simulink model "complete_plant"  (R2021b)
settings: Solver=VariableStepAuto  StartTime=0.0  StopTime=15  RelTol=1e-3
values from neighbouring files (symbols this model uses):
  a = Simulink.Parameter(1.14)    [startup.m]
  A1 = Simulink.Parameter(39.8344)    [startup.m]
  A2 = Simulink.Parameter(813.0780)    [startup.m]
  b = Simulink.Parameter(-0.03291)    [startup.m]
  B1 = Simulink.Parameter(0.000001287)    [startup.m]
  B2 = Simulink.Parameter(-0.002325)    [startup.m]
  B3 = Simulink.Parameter(3.797)    [startup.m]
  c = Simulink.Parameter(-1.14)    [startup.m]
  C1 = Simulink.Parameter(-0.000000002541)    [startup.m]
  C2 = Simulink.Parameter(0.000005279)    [startup.m]
  C3 = Simulink.Parameter(-0.003943)    [startup.m]
  C4 = Simulink.Parameter(3.634)    [startup.m]
  C_param = Simulink.Parameter([0 13757.41 21278.97 26666.02 30253.47 30313.18 30313.18])    [startup.m]
  d = Simulink.Parameter(-1.027)    [startup.m]
  driver_gain = 1    [startup.m]
  FZ_C = Simulink.Parameter([0 204.13 427.04 668.1 895.72 1124.40 1324.40])    [startup.m]
  gr = Simulink.Parameter([6.63043, 6.63043, 7.95652, 7.95652])    [startup.m]
  I = 15    [startup.m]
  inch2mm = Simulink.Parameter(25.4)    [startup.m]
  J_z = Simulink.Parameter(75)    [startup.m]
  k_limit = Simulink.Parameter(3.461)    [startup.m]
  Ku = Simulink.Parameter(0.24 / g.Value)    [startup.m]
  l = Simulink.Parameter([0.7922471, 0.7828529])    [startup.m]
  max_yaw_field = Simulink.Parameter([1.34 1.34 1.34 1.66 1.14 1.24 0.754 0.849 0.85 0.85])    [startup.m]
  min_speed_regen = Simulink.Parameter(85)    [startup.m]
  motor_efficiency = Simulink.Parameter([0.85, 0.85, 0.85, 0.85])    [startup.m]
  motor_limit_power = Simulink.Parameter([15000, 15000, 15000, 15000])    [startup.m]
  motor_limit_torque = Simulink.Parameter([-25, 25])    [startup.m]
  mu_factor = Simulink.Parameter(2/3)    [startup.m]
  P = 1    [startup.m]
  ramp_rate = 1    [startup.m]
  RE = Simulink.Parameter(0.2228169203)    [startup.m]
  s = Simulink.Parameter([0.647895, 0.62102])    [startup.m]
  S1 = Simulink.Parameter(7 * (10^(-5)))    [startup.m]
  S2 = Simulink.Parameter(-0.0038)    [startup.m]
  S3 = Simulink.Parameter(0.6535)    [startup.m]
  S4 = Simulink.Parameter(0.1061)    [startup.m]
  steer_slope = Simulink.Parameter(0.0111)    [startup.m]
  T = 0    [startup.m]
  T2F = Simulink.Parameter(single([29 29 35 35]))    [startup.m]
  tau = Simulink.Parameter(0)    [startup.m]
  time_delay = 0.022    [startup.m]
  V_target = Simulink.Parameter([0 3 6 9 12 15 18 21 25 31])    [startup.m]
undefined symbols (not defined in the file or in its folder): DiscIntNeverNeededParam
libraries: fl_lib x20, nesl_utility x12, sdl_lib x4, slpidlib x2, simulink x2, autolibdatasheetbattery x1, autolibmappedmotor x1, vehdynlibtire x1, autolibshared x1, vehdynlibviscommon x1
(part 1 of 4)
settings Model: Creator=Inver  LastModifiedBy=Inver
settings DataIOCC: ExternalInput=straight_accel.getElement('driver_input'),straight_accel.getElement('P_A'),straight_accel.getElement('B_A'),straight_accel.getElement('steering_angle'),straight_accel.getElement('batt_temp'),straight_accel.getElement('pressure_front'),straight_accel.getElement('pressure_rear')  LoadExternalInput=on
settings OptimizationCC: DefaultParameterBehavior=Inlined  UseDivisionForNetSlopeComputation=on  GainParamInheritBuiltInType=on  UseFloatMulNetSlope=on  InlineInvariantSignals=on  PassReuseOutputArgsAs=Individual arguments  ZeroExternalMemoryAtStartup=off  ZeroInternalMemoryAtStartup=off  NoFixptDivByZeroProtection=on  EfficientFloat2IntCast=on  LifeSpan=1  OptimizeBlockOrder=speed  DifferentSizesBufferReuse=on  EfficientTunableParamExpr=on
settings DebuggingCC: ParameterTunabilityLossMsg=error
settings HardwareCC: ProdBitPerPointer=32  ProdBitPerSizeT=32  ProdBitPerPtrDiffT=32  ProdLargestAtomicInteger=Long  ProdLargestAtomicFloat=Double  ProdWordSize=32  ProdLongLongMode=on  ProdHWDeviceType=ARM Compatible->ARM Cortex-M
settings SFSimCC: SimCustomHeaderCode="#include \"bigM_v2_func.h\""  SimUserSources=bigM_v2_func.c  MATLABDynamicMemAlloc=off
settings RTWCC: Description=Embedded Coder  SystemTargetFile=ert.tlc  GenCodeOnly=on  TemplateMakefile=ert_default_tmf  BuildConfiguration=Faster Runs
settings CodeAppCC: ForceParamTrailComments=on  IgnoreCustomStorageClasses=off  OperatorAnnotations=on  SimulinkDataObjDesc=on  SFDataObjDesc=on  CustomSymbolStrGlobalVar=rt$N$M  CustomSymbolStrType=$N$M  CustomSymbolStrFcn=$N$M$F  CustomSymbolStrMacro=$N$M  InsertBlockDesc=on
settings ERTTargetCC: TargetLangStandard=C99 (ISO)  GenerateSampleERTMain=on  IncludeMdlTerminateFcn=off  CombineSignalStateStructs=on  SupportComplex=off  SupportNonInlinedSFcns=on  InlinedParameterPlacement=NonHierarchical  ERTCustomFileTemplate=example_file_process.tlc  ERTFilePackagingFormat=CompactWithDataFile

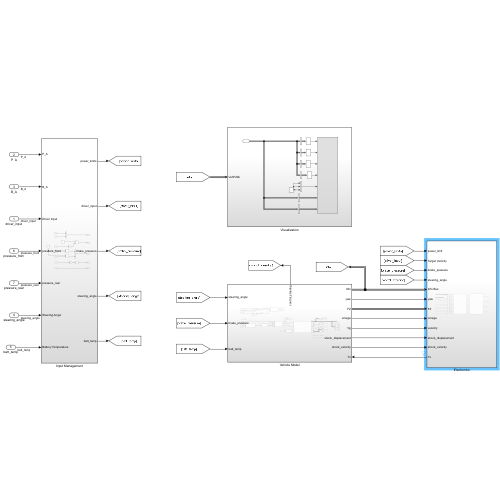
[thumbnail: Simulink's stored preview of the top-level diagram]
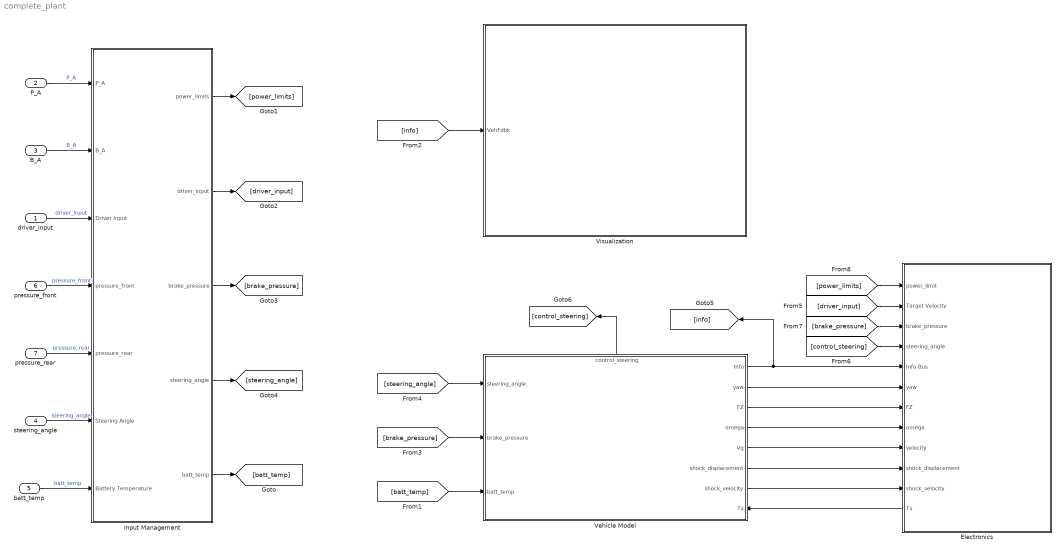
== system complete_plant ==
  driver_input : Inport  Interpolate=off
  P_A : Inport  Port=2  Interpolate=off
  B_A : Inport  Port=3  Interpolate=off
  steering_angle : Inport  Port=4
  batt_temp : Inport  Port=5  Interpolate=off
  pressure_front : Inport  Port=6  Interpolate=off
  pressure_rear : Inport  Port=7  Interpolate=off
  Electronics : Subsystem
      settings: PortSchema="{\"entries\":[{\"content\":{\"sides\":[{\"content\":{\"connectorIds\":[\"In1\",\"In2\",\"In3\",\"In4\",\"In5\",\"In6\",\"In7\",\"In8\",\"In9\",\"In10\",\"In11\",\"Out1\"]},\"type\":\"ConnectorPlacement.EquallySpacedRectSide\",\"uuid\":\"60aa76ce-4868-40a7-a4fe-105a8e1f1745\"},{\"content\":{\"connectorIds\":[],\"side\":\"RIGHT\"},\"type\":\"ConnectorPlacement.EquallySpacedRectSide\",\"uuid\":\"32a33737-884d-4b24-9f96-3d3edd17fbca\"},{\"content\":{\"connectorIds\":[],\"side\":\"TOP\"},\"type\":\"ConnectorPlacement.EquallySpacedRectSide\",\"uuid\":\"827704d2-5b88-4535-b448-6dd72aa29b4b\"},{\"content\":{\"connectorIds\":[],\"side\":\"BOTTOM\"},\"type\":\"ConnectorPlacement.EquallySpacedRectSide\",\"uuid\":\"278cc67c-48ea-4083-b722-927ef88660f9\"},{\"content\":{\"connectorIds\":[],\"side\":\"HIDDEN\"},\"type\":\"ConnectorPlacement.EquallySpacedRectSide\",\"uuid\":\"0c403b58-0099-4716-b0b3-86e3ff44a502\"}]},\"type\":\"ConnectorPlacement.EquallySpacedConnector\",\"uuid\":\"f0e3ee49-9104-4d68-bbfb-d96c82f46588\"}],\"packageUris\":[\"http://schema.mathworks.com/mf0/Connector/R2020b\"],\"version\":\"1.0\"}"
  Input Management : Subsystem
  Vehicle Model : Subsystem
      settings: PortSchema="{\"entries\":[{\"content\":{\"sides\":[{\"content\":{\"connectorIds\":[\"In1\",\"In2\",\"In3\"]},\"type\":\"ConnectorPlacement.EquallySpacedRectSide\",\"uuid\":\"7263df3d-11c2-488e-998f-6bd776306b9c\"},{\"content\":{\"connectorIds\":[\"Out1\",\"Out2\",\"Out3\",\"Out4\",\"Out5\",\"Out6\",\"Out7\",\"In4\"],\"side\":\"RIGHT\"},\"type\":\"ConnectorPlacement.EquallySpacedRectSide\",\"uuid\":\"b0de89c2-35d2-4c59-81fc-f1f509ccf522\"},{\"content\":{\"connectorIds\":[\"Out8\"],\"side\":\"TOP\"},\"type\":\"ConnectorPlacement.EquallySpacedRectSide\",\"uuid\":\"474ba072-8402-41d1-8015-97ca573757b9\"}]},\"type\":\"ConnectorPlacement.EquallySpacedConnector\",\"uuid\":\"426f55ca-7f3f-41f0-94e6-91e6d6304a5e\"}],\"packageUris\":[\"http://schema.mathworks.com/mf0/Connector/R2020b\"],\"version\":\"1.0\"}"
  Visualization : Subsystem
  wires:
  Vehicle Model/5(Vg) -> Electronics/9(velocity)
  Vehicle Model/4(omega) -> Electronics/8(omega)
  [brake_pressure] -> Vehicle Model/2(brake_pressure)
  Vehicle Model/1(Info) -> [info], Electronics/5(Info Bus)
  Vehicle Model/3(FZ) -> Electronics/7(FZ)
  Vehicle Model/2(yaw) -> Electronics/6(yaw)
  Vehicle Model/6(shock_displacement) -> Electronics/10(shock_displacement)
  Vehicle Model/7(shock_velocity) -> Electronics/11(shock_velocity)
  [batt_temp] -> Vehicle Model/3(batt_temp)
  steering_angle/1 -> Input Management/6(Steering Angle)  "steering_angle"
  driver_input/1 -> Input Management/3(Driver Input)  "driver_input"
  P_A/1 -> Input Management/1(P_A)  "P_A"
  pressure_front/1 -> Input Management/4(pressure_front)  "pressure_front"
  B_A/1 -> Input Management/2(B_A)  "B_A"
  pressure_rear/1 -> Input Management/5(pressure_rear)  "pressure_rear"
  batt_temp/1 -> Input Management/7(Battery Temperature)  "batt_temp"
  Input Management/5(batt_temp) -> [batt_temp]
  Input Management/4(steering_angle) -> [steering_angle]
  Input Management/3(brake_pressure) -> [brake_pressure]
  Input Management/2(driver_input) -> [driver_input]
  Input Management/1(power_limits) -> [power_limits]
  [power_limits] -> Electronics/1(power_limit)
  [driver_input] -> Electronics/2(Target Velocity)
  [brake_pressure] -> Electronics/3(brake_pressure)
  [control_steering] -> Electronics/4(steering_angle)
  [steering_angle] -> Vehicle Model/1(steering_angle)
  [info] -> Visualization/1(VehFdbk)
  Electronics/1(Tx) -> Vehicle Model/4(Tx)
  Vehicle Model/8(control_steering) -> [control_steering]

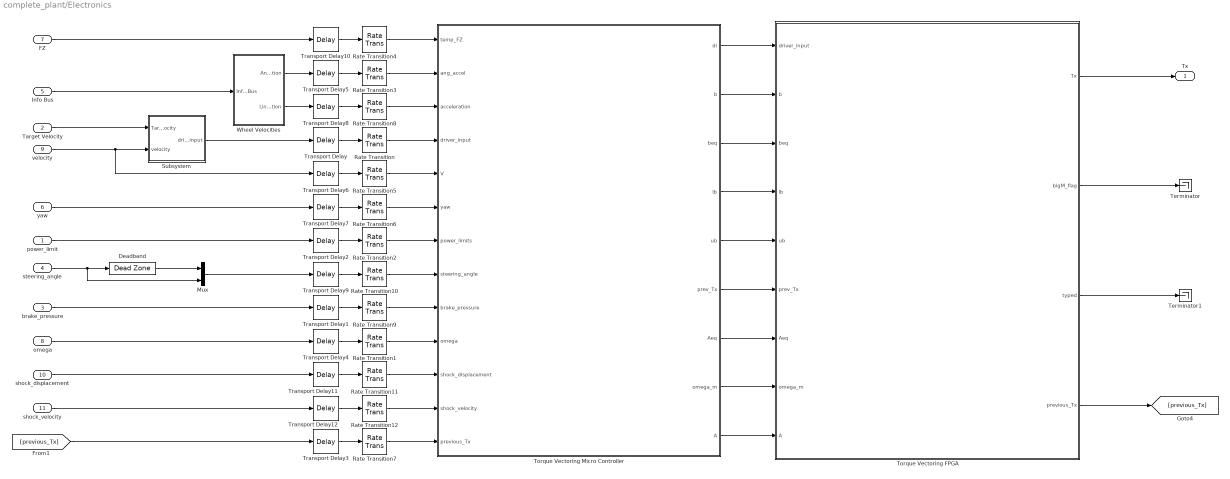
== system complete_plant/Electronics ==
  power_limit : Inport
  Target Velocity : Inport  Port=2
  brake_pressure : Inport  Port=3  PortDimensions=[1 4]
  steering_angle : Inport  Port=4
  Info Bus : Inport  Port=5
  yaw : Inport  Port=6
  FZ : Inport  Port=7
  omega : Inport  Port=8
  velocity : Inport  Port=9
  shock_displacement : Inport  Port=10
  shock_velocity : Inport  Port=11
  " Wheel Velocities" : Subsystem
  Deadband : DeadZone  LowerValue=-3  UpperValue=3  SaturateOnIntegerOverflow=on
  Mux : Mux  Inputs=2
  Rate Transition : RateTransition  OutPortSampleTime=0.015
  Rate Transition{1,7,9,11..12} (5 alike) : RateTransition  InitialCondition=[0 0 0 0]  OutPortSampleTime=0.015
  Rate Transition{2,5,8,10} (4 alike) : RateTransition  InitialCondition=[0 0]  OutPortSampleTime=0.015
  Rate Transition3 : RateTransition  OutPortSampleTime=0.015
  Rate Transition4 : RateTransition  InitialCondition=[450 450 450 450]  OutPortSampleTime=0.015
  Rate Transition6 : RateTransition  OutPortSampleTime=0.015
  Subsystem : Subsystem
  Terminator : Terminator
  Terminator1 : Terminator
  Torque Vectoring FPGA : Subsystem
  Torque Vectoring Micro Controller : Subsystem
  Transport Delay : TransportDelay  DelayTime=time_delay  BufferSize=25000
  Transport Delay{1,3..4,11..12} (5 alike) : TransportDelay  DelayTime=time_delay  InitialOutput=[0 0 0 0]  BufferSize=25000
  Transport Delay10 : TransportDelay  DelayTime=time_delay  InitialOutput=[450 450 450 450]  BufferSize=25000
  Transport Delay{2,6,8..9} (4 alike) : TransportDelay  DelayTime=time_delay  InitialOutput=[0 0]  BufferSize=25000
  Transport Delay5 : TransportDelay  DelayTime=time_delay  BufferSize=25000
  Transport Delay7 : TransportDelay  DelayTime=time_delay  BufferSize=25000
  Tx : Outport  PortDimensions=[1 4]
  wires:
  Info Bus/1 -> " Wheel Velocities"/1(Info Bus)
  Transport Delay6/1 -> Rate Transition5/1
  Transport Delay2/1 -> Rate Transition2/1
  power_limit/1 -> Transport Delay2/1
  Transport Delay7/1 -> Rate Transition6/1
  Transport Delay10/1 -> Rate Transition4/1
  FZ/1 -> Transport Delay10/1
  Subsystem/1(driver_input) -> Transport Delay/1
  yaw/1 -> Transport Delay7/1
  velocity/1 -> Transport Delay6/1, Subsystem/2(velocity)
  Target Velocity/1 -> Subsystem/1(Target Velocity)
  Rate Transition4/1 -> Torque Vectoring Micro Controller/1(temp_FZ)
  Rate Transition6/1 -> Torque Vectoring Micro Controller/6(yaw)
  Rate Transition/1 -> Torque Vectoring Micro Controller/4(driver_input)
  Transport Delay1/1 -> Rate Transition9/1
  brake_pressure/1 -> Transport Delay1/1
  Transport Delay9/1 -> Rate Transition10/1
  Rate Transition10/1 -> Torque Vectoring Micro Controller/8(steering_angle)
  Torque Vectoring FPGA/2(bigM_flag) -> Terminator/1
  Torque Vectoring FPGA/3(typed) -> Terminator1/1
  Rate Transition5/1 -> Torque Vectoring Micro Controller/5(V)
  Rate Transition2/1 -> Torque Vectoring Micro Controller/7(power_limits)
  Transport Delay5/1 -> Rate Transition3/1
  Rate Transition3/1 -> Torque Vectoring Micro Controller/2(ang_accel)
  " Wheel Velocities"/1(Angular Acceleration) -> Transport Delay5/1
  Transport Delay/1 -> Rate Transition/1
  Transport Delay4/1 -> Rate Transition1/1
  Transport Delay11/1 -> Rate Transition11/1
  Transport Delay12/1 -> Rate Transition12/1
  omega/1 -> Transport Delay4/1
  shock_displacement/1 -> Transport Delay11/1
  shock_velocity/1 -> Transport Delay12/1
  Torque Vectoring FPGA/1(Tx) -> Tx/1
  Torque Vectoring Micro Controller/1(di) -> Torque Vectoring FPGA/1(driver_input)
  Torque Vectoring Micro Controller/2(b) -> Torque Vectoring FPGA/2(b)
  Torque Vectoring Micro Controller/3(beq) -> Torque Vectoring FPGA/3(beq)
  Torque Vectoring Micro Controller/4(lb) -> Torque Vectoring FPGA/4(lb)
  Torque Vectoring Micro Controller/8(omega_m) -> Torque Vectoring FPGA/8(omega_m)
  Torque Vectoring Micro Controller/7(Aeq) -> Torque Vectoring FPGA/7(Aeq)
  Torque Vectoring Micro Controller/6(prev_Tx) -> Torque Vectoring FPGA/6(prev_Tx)
  Torque Vectoring Micro Controller/9(A) -> Torque Vectoring FPGA/9(A)
  Torque Vectoring FPGA/4(previous_Tx) -> [previous_Tx]
  Transport Delay3/1 -> Rate Transition7/1
  [previous_Tx] -> Transport Delay3/1
  Rate Transition9/1 -> Torque Vectoring Micro Controller/9(brake_pressure)
  Rate Transition1/1 -> Torque Vectoring Micro Controller/10(omega)
  Rate Transition11/1 -> Torque Vectoring Micro Controller/11(shock_displacement)
  Rate Transition12/1 -> Torque Vectoring Micro Controller/12(shock_velocity)
  Rate Transition7/1 -> Torque Vectoring Micro Controller/13(previous_Tx)
  Torque Vectoring Micro Controller/5(ub) -> Torque Vectoring FPGA/5(ub)
  Transport Delay8/1 -> Rate Transition8/1
  Rate Transition8/1 -> Torque Vectoring Micro Controller/3(acceleration)
  " Wheel Velocities"/2(Linear Acceleration) -> Transport Delay8/1
  steering_angle/1 -> Mux/2, Deadband/1
  Deadband/1 -> Mux/1
  Mux/1 -> Transport Delay9/1

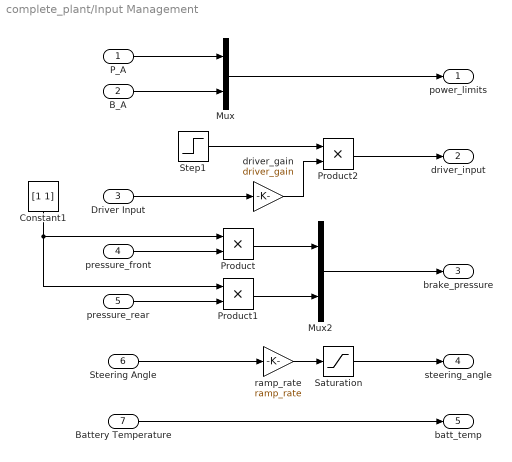
== system complete_plant/Input Management ==
  P_A : Inport
  B_A : Inport  Port=2
  Driver Input : Inport  Port=3
  pressure_front : Inport  Port=4
  pressure_rear : Inport  Port=5
  Steering Angle : Inport  Port=6
  Battery Temperature : Inport  Port=7
  Constant1 : Constant  Value=[1 1]  VectorParams1D=off
  Mux : Mux  Inputs=2
  Mux2 : Mux  Inputs=2
  Product : Product
  Product1 : Product
  Product2 : Product
  Saturation : Saturate  UpperLimit=30  LowerLimit=-30
  Step1 : Step  Time=0.05  SampleTime=0
  driver_gain : Gain  Gain=driver_gain
  ramp_rate : Gain  Gain=ramp_rate
  power_limits : Outport
  driver_input : Outport  Port=2
  brake_pressure : Outport  Port=3
  steering_angle : Outport  Port=4
  batt_temp : Outport  Port=5
  wires:
  ramp_rate/1 -> Saturation/1
  Steering Angle/1 -> ramp_rate/1
  Driver Input/1 -> driver_gain/1
  Mux/1 -> power_limits/1
  P_A/1 -> Mux/1
  B_A/1 -> Mux/2
  Saturation/1 -> steering_angle/1
  pressure_front/1 -> Product/2
  Battery Temperature/1 -> batt_temp/1
  Product/1 -> Mux2/1
  Product1/1 -> Mux2/2
  Mux2/1 -> brake_pressure/1
  Constant1/1 -> Product1/1, Product/1
  pressure_rear/1 -> Product1/2
  Step1/1 -> Product2/1
  driver_gain/1 -> Product2/2
  Product2/1 -> driver_input/1

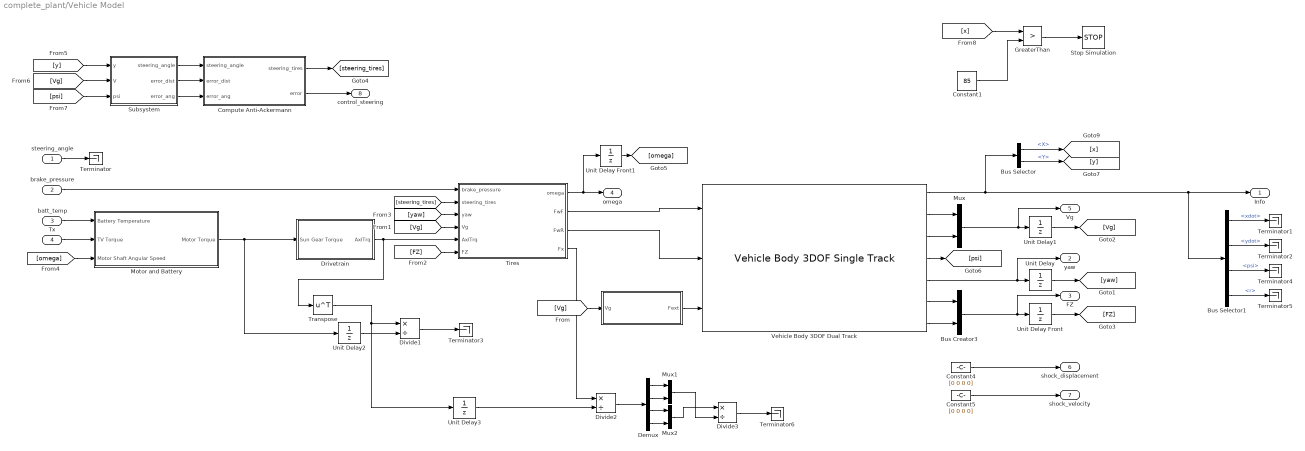
== system complete_plant/Vehicle Model ==
  steering_angle : Inport
  brake_pressure : Inport  Port=2
  batt_temp : Inport  Port=3
  Tx : Inport  Port=4
  "  " : MATLAB Function  TreatAsAtomicUnit=on  SystemSampleTime=0.0005
  Bus Creator3 : BusCreator  Inputs=2
  Bus Selector : BusSelector  OutputSignals=InertFrm.Cg.Disp.X,InertFrm.Cg.Disp.Y
  Bus Selector1 : BusSelector  OutputSignals=BdyFrm.Cg.Vel.xdot,BdyFrm.Cg.Vel.ydot,InertFrm.Cg.Ang.psi,BdyFrm.Cg.AngVel.r
  Compute Anti-Ackermann : MATLAB Function  TreatAsAtomicUnit=on  SystemSampleTime=0.0005
  Constant1 : Constant  Value=85
  Constant4 : Constant  Value=[0 0 0 0]
  Constant5 : Constant  Value=[0 0 0 0]
  Demux : Demux
  Divide1 : Product  Inputs=*/
  Divide2 : Product  Inputs=*/
  Divide3 : Product  Inputs=*/
  Drivetrain : Subsystem
  GreaterThan : RelationalOperator  Operator=>  OutDataTypeStr=boolean  RndMeth=Simplest
  Motor and Battery : Subsystem
      settings: PortSchema="{\"entries\":[{\"content\":{\"sides\":[{\"content\":{\"connectorIds\":[\"Out1\"]},\"type\":\"ConnectorPlacement.EquallySpacedRectSide\",\"uuid\":\"0a1f914b-70eb-46fa-9e3d-552685e5145b\"},{\"content\":{\"connectorIds\":[\"In1\",\"In2\",\"In3\"],\"side\":\"RIGHT\"},\"type\":\"ConnectorPlacement.EquallySpacedRectSide\",\"uuid\":\"3f4913ad-53b1-4c2d-9942-63851d66d84d\"},{\"content\":{\"connectorIds\":[],\"side\":\"TOP\"},\"type\":\"ConnectorPlacement.EquallySpacedRectSide\",\"uuid\":\"355326fa-9c02-45e7-a319-d2a0d6b3d4bd\"},{\"content\":{\"connectorIds\":[],\"side\":\"HIDDEN\"},\"type\":\"ConnectorPlacement.EquallySpacedRectSide\",\"uuid\":\"65af7ff0-f0aa-4be0-a188-dc3dcb8956e6\"}]},\"type\":\"ConnectorPlacement.EquallySpacedConnector\",\"uuid\":\"023a46d9-a637-4c8e-84c1-6893dcef87c2\"}],\"packageUris\":[\"http://schema.mathworks.com/mf0/Connector/R2020b\"],\"version\":\"1.0\"}"
  Mux : Mux  Inputs=2
  Mux1 : Mux  Inputs=2
  Mux2 : Mux  Inputs=2
  Stop Simulation : Stop
  Subsystem : Subsystem
  Terminator{,1..6} (7 alike) : Terminator
  Tires : Subsystem
  Transpose : Math  Operator=transpose  SaturateOnIntegerOverflow=on
  Unit Delay : UnitDelay  SampleTime=0.0005  HasFrameUpgradeWarning=on
  Unit Delay Front : UnitDelay  InitialCondition=[450 450 450 450]  SampleTime=0.0005  HasFrameUpgradeWarning=on
  Unit Delay Front1 : UnitDelay  InitialCondition=[0 0 0 0]  SampleTime=0.0005  HasFrameUpgradeWarning=on
  Unit Delay1 : UnitDelay  InitialCondition=[0.1 0.1]  SampleTime=0.0005  HasFrameUpgradeWarning=on
  Unit Delay2 : UnitDelay  InitialCondition=[0 0 0 0]  SampleTime=0.0005  HasFrameUpgradeWarning=on
  Unit Delay3 : UnitDelay  InitialCondition=[0 0 0 0]  SampleTime=0.0005  HasFrameUpgradeWarning=on
  Vehicle Body 3DOF Dual Track : autolibshared/Vehicle Body 3DOF Single Track  trackMode=Dual  inputMode=External forces  frontSteerMode=off  rearSteerMode=off  windMode=off  muMode=off  extFMode=on  extMMode=off  htchFMode=off  htchMMode=off  extXo=off  extpsio=off  extxdoto=off  extro=off  extYo=off  extTamb=off  extydoto=off  aMode=2  NF=2  NR=2  m=308  a=0.7922471  b=0.7828529  h=0.295  dh=1  hh=0.2  X_o=0  xdot_o=0  CalphaMode=off  sigmaMode=on  d=0  hl=0  w=[1.29579,1.24204]  Cy_f=25e3  Cy_r=25e3  sigma_f=.1  sigma_r=.1  alpha_f_brk=[-.1 .1]  Cy_f_data=[-9e3 9e3]  alpha_r_brk=[-.1 .1]  Cy_r_data=[-9e3 9e3]  Y_o=0  ydot_o=0  Izz=200  psi_o=0  r_o=0  Af=1.0221  Cd=1.149  Cl=0  Cpm=.00000001  beta_w=[0:0.01:0.1]  Cs=[0:0.0000001:0.000001]  Cym=[0:0.0000001:0.000001]  Pabs=101325  Tair=273  g=9.81  mu=1  xdot_tol=.001  Fznom=15000  Fxtire_sat=7e4  Fytire_sat=7e4  longOff=0  latOff=0  vertOff=0  wrapAng=off
      settings: SourceProductBaseCode=PW,DR,MT,UV,VE
  Info : Outport
  yaw : Outport  Port=2
  FZ : Outport  Port=3
  omega : Outport  Port=4
  Vg : Outport  Port=5
  shock_displacement : Outport  Port=6
  shock_velocity : Outport  Port=7
  control_steering : Outport  Port=8
  wires:
  Vehicle Body 3DOF Dual Track/1 -> Bus Selector/1, Bus Selector1/1, Info/1
  Bus Selector/1 -> [x]  "<X>"
  Bus Selector/2 -> [y]  "<Y>"
  Vehicle Body 3DOF Dual Track/7 -> Bus Creator3/2
  Vehicle Body 3DOF Dual Track/6 -> Bus Creator3/1
  "  "/1(Fext) -> Vehicle Body 3DOF Dual Track/3
  Bus Creator3/1 -> Unit Delay Front/1, FZ/1
  Vehicle Body 3DOF Dual Track/3 -> Mux/2
  Vehicle Body 3DOF Dual Track/2 -> Mux/1
  Mux/1 -> Unit Delay1/1, Vg/1
  Vehicle Body 3DOF Dual Track/5 -> Unit Delay/1, yaw/1
  Unit Delay1/1 -> [Vg]
  Unit Delay/1 -> [yaw]
  [Vg] -> "  "/1(Vg)
  Unit Delay Front/1 -> [FZ]
  brake_pressure/1 -> Tires/1(brake_pressure)
  Tires/1(omega) -> omega/1, Unit Delay Front1/1
  [FZ] -> Tires/6(FZ)
  [steering_tires] -> Tires/2(steering_tires)
  Tires/2(FwF) -> Vehicle Body 3DOF Dual Track/1
  Tires/3(FwR) -> Vehicle Body 3DOF Dual Track/2
  [Vg] -> Tires/4(Vg)
  [yaw] -> Tires/3(yaw)
  Constant5/1 -> shock_velocity/1
  Constant4/1 -> shock_displacement/1
  Unit Delay Front1/1 -> [omega]
  [omega] -> Motor and Battery/1(Motor Shaft Angular Speed)
  batt_temp/1 -> Motor and Battery/3(Battery Temperature)
  Vehicle Body 3DOF Dual Track/4 -> [psi]
  Motor and Battery/1(Motor Torque) -> Drivetrain/1(Sun Gear Torque), Unit Delay2/1
  steering_angle/1 -> Terminator/1
  Bus Selector1/1 -> Terminator1/1  "<xdot>"
  Bus Selector1/2 -> Terminator2/1  "<ydot>"
  Bus Selector1/3 -> Terminator4/1  "<psi>"
  Bus Selector1/4 -> Terminator5/1  "<r>"
  Tx/1 -> Motor and Battery/2(TV Torque)
  Compute Anti-Ackermann/1(steering_tires) -> [steering_tires]
  Compute Anti-Ackermann/2(error) -> control_steering/1
  GreaterThan/1 -> Stop Simulation/1
  [x] -> GreaterThan/1
  Constant1/1 -> GreaterThan/2
  Divide1/1 -> Terminator3/1
  Divide2/1 -> Demux/1
  Tires/4(Fx) -> Divide2/1
  Demux/1 -> Mux1/1
  Demux/2 -> Mux1/2
  Demux/4 -> Mux2/2
  Demux/3 -> Mux2/1
  Mux1/1 -> Divide3/2
  Mux2/1 -> Divide3/1
  Divide3/1 -> Terminator6/1
  Transpose/1 -> Unit Delay3/1, Divide1/1
  Drivetrain/1(AxlTrq) -> Transpose/1, Tires/5(AxlTrq)
  Unit Delay2/1 -> Divide1/2
  Unit Delay3/1 -> Divide2/2
  [y] -> Subsystem/1(y)
  [Vg] -> Subsystem/2(V)
  [psi] -> Subsystem/3(psi)
  Subsystem/1(steering_angle) -> Compute Anti-Ackermann/1(steering_angle)
  Subsystem/2(error_dist) -> Compute Anti-Ackermann/2(error_dist)
  Subsystem/3(error_ang) -> Compute Anti-Ackermann/3(error_ang)

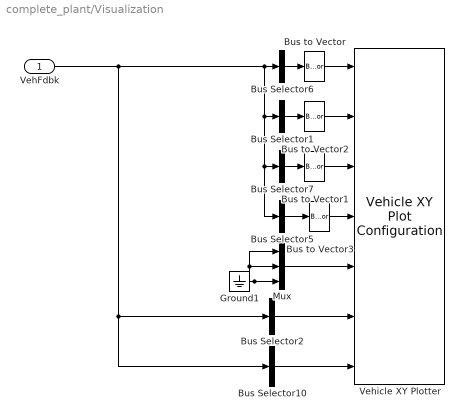
== system complete_plant/Visualization ==
  VehFdbk : Inport
  Bus Selector1 : BusSelector  OutputSignals=InertFrm.Cg.Ang.phi,InertFrm.Cg.Ang.theta,InertFrm.Cg.Ang.psi  OutputAsBus=on
  Bus Selector10 : BusSelector  OutputSignals=BdyFrm.Forces.FrntAxl.Lft.Fy,BdyFrm.Forces.FrntAxl.Rght.Fy,BdyFrm.Forces.RearAxl.Lft.Fy,BdyFrm.Forces.RearAxl.Rght.Fy  OutputAsBus=on
  Bus Selector2 : BusSelector  OutputSignals=BdyFrm.Forces.FrntAxl.Lft.Fx,BdyFrm.Forces.FrntAxl.Rght.Fx,BdyFrm.Forces.RearAxl.Lft.Fx,BdyFrm.Forces.RearAxl.Rght.Fx  OutputAsBus=on
  Bus Selector5 : BusSelector  OutputSignals=BdyFrm.FrntAxl.Steer.WhlAngFL,BdyFrm.FrntAxl.Steer.WhlAngFR,BdyFrm.RearAxl.Steer.WhlAngRL,BdyFrm.RearAxl.Steer.WhlAngRR  OutputAsBus=on
  Bus Selector6 : BusSelector  OutputSignals=InertFrm.Cg.Disp.X,InertFrm.Cg.Disp.Y,InertFrm.Cg.Disp.Z  OutputAsBus=on
  Bus Selector7 : BusSelector  OutputSignals=InertFrm.Cg.Vel.Xdot,InertFrm.Cg.Vel.Ydot,InertFrm.Cg.Vel.Zdot  OutputAsBus=on
  Bus to Vector{,1..3} (4 alike) : BusToVector
  Ground1 : Ground
  Mux : Mux  Inputs=3
  Vehicle XY Plotter : vehdynlibviscommon/Vehicle XY Plot Configuration  extRef=on  extStats=off  extTireF=on  a=0.7922471  b=0.7828529  w=1.26  figBorder=10  bufferSize=1024  velNorm=5  tireFNorm=1000  pltDT=.1
      settings: SourceProductBaseCode=VE
  wires:
  Bus Selector1/1 -> Bus to Vector2/1
  VehFdbk/1 -> Bus Selector2/1, Bus Selector10/1, Bus Selector5/1, Bus Selector7/1, Bus Selector1/1, Bus Selector6/1
  Mux/1 -> Vehicle XY Plotter/5
  Bus Selector7/1 -> Bus to Vector1/1
  Bus to Vector2/1 -> Vehicle XY Plotter/2
  Bus to Vector1/1 -> Vehicle XY Plotter/3
  Bus Selector6/1 -> Bus to Vector/1
  Bus to Vector/1 -> Vehicle XY Plotter/1
  Ground1/1 -> Mux/3, Mux/2, Mux/1
  Bus Selector2/1 -> Vehicle XY Plotter/6
  Bus Selector10/1 -> Vehicle XY Plotter/7
  Bus to Vector3/1 -> Vehicle XY Plotter/4
  Bus Selector5/1 -> Bus to Vector3/1

== system complete_plant/Electronics/ Wheel Velocities ==
  Info Bus : Inport
  Bus Selector1 : BusSelector  OutputSignals=BdyFrm.Cg.AngAcc.rdot,BdyFrm.Cg.Acc.xddot,BdyFrm.Cg.Acc.yddot
  Mux : Mux  Inputs=2
  Angular Acceleration : Outport
  Linear Acceleration : Outport  Port=2
  wires:
  Info Bus/1 -> Bus Selector1/1
  Bus Selector1/1 -> Angular Acceleration/1  "<rdot>"
  Bus Selector1/3 -> Mux/2  "<yddot>"
  Bus Selector1/2 -> Mux/1  "<xddot>"
  Mux/1 -> Linear Acceleration/1

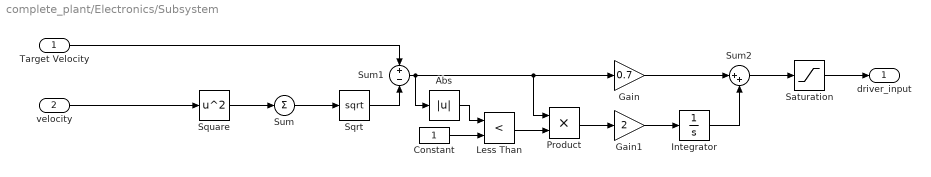
== system complete_plant/Electronics/Subsystem ==
  Target Velocity : Inport
  velocity : Inport  Port=2
  Abs : Abs
  Constant : Constant
  Gain : Gain  Gain=0.7
  Gain1 : Gain  Gain=2
  Integrator : Integrator  LimitOutput=on  UpperSaturationLimit=1  LowerSaturationLimit=-1
  Less Than : RelationalOperator  Operator=<  OutDataTypeStr=boolean  RndMeth=Simplest
  Product : Product
  Saturation : Saturate  UpperLimit=1  LowerLimit=-1
  Sqrt : Sqrt  SaturateOnIntegerOverflow=on
  Square : Math  Operator=square  SaturateOnIntegerOverflow=on
  Sum : Sum  Inputs=+
  Sum1 : Sum  Inputs=+-
  Sum2 : Sum  Inputs=|++
  driver_input : Outport
  wires:
  Target Velocity/1 -> Sum1/1
  Sqrt/1 -> Sum1/2
  Square/1 -> Sum/1
  Sum/1 -> Sqrt/1
  velocity/1 -> Square/1
  Gain1/1 -> Integrator/1
  Gain/1 -> Sum2/1
  Integrator/1 -> Sum2/2
  Product/1 -> Gain1/1
  Sum2/1 -> Saturation/1
  Saturation/1 -> driver_input/1
  Less Than/1 -> Product/2
  Constant/1 -> Less Than/2
  Abs/1 -> Less Than/1
  Sum1/1 -> Gain/1, Product/1, Abs/1

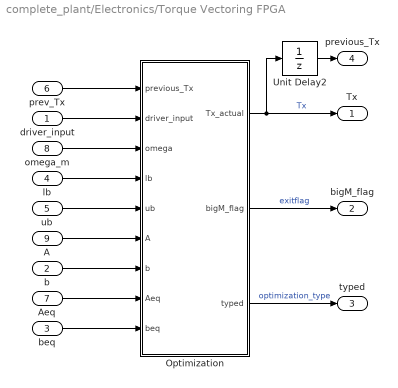
== system complete_plant/Electronics/Torque Vectoring FPGA ==
  driver_input : Inport  PortDimensions=1
  b : Inport  Port=2  PortDimensions=1
  beq : Inport  Port=3  PortDimensions=1
  lb : Inport  Port=4  PortDimensions=[1 4]
  ub : Inport  Port=5  PortDimensions=[1 4]
  prev_Tx : Inport  Port=6  PortDimensions=[1 4]
  Aeq : Inport  Port=7  PortDimensions=[1 4]
  omega_m : Inport  Port=8  PortDimensions=[1 4]
  A : Inport  Port=9  PortDimensions=[1 4]
  "Optimization " : MATLAB Function  TreatAsAtomicUnit=on
  Unit Delay2 : UnitDelay  SampleTime=-1  HasFrameUpgradeWarning=on
  Tx : Outport  PortDimensions=[1 4]
  bigM_flag : Outport  Port=2  PortDimensions=1
  typed : Outport  Port=3  PortDimensions=1
  previous_Tx : Outport  Port=4  PortDimensions=[1 4]
  wires:
  "Optimization "/1(Tx_actual) -> Tx/1, Unit Delay2/1  "Tx"
  "Optimization "/2(bigM_flag) -> bigM_flag/1  "exitflag"
  b/1 -> "Optimization "/7(b)
  prev_Tx/1 -> "Optimization "/1(previous_Tx)
  "Optimization "/3(typed) -> typed/1  "optimization_type"
  driver_input/1 -> "Optimization "/2(driver_input)
  omega_m/1 -> "Optimization "/3(omega)
  beq/1 -> "Optimization "/9(beq)
  lb/1 -> "Optimization "/4(lb)
  ub/1 -> "Optimization "/5(ub)
  A/1 -> "Optimization "/6(A)
  Aeq/1 -> "Optimization "/8(Aeq)
  Unit Delay2/1 -> previous_Tx/1

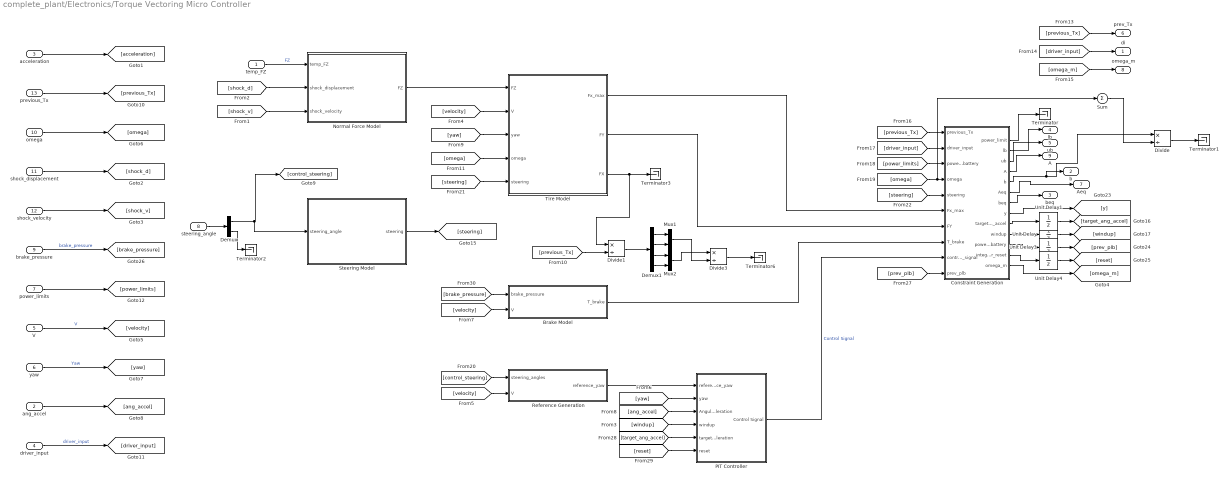
== system complete_plant/Electronics/Torque Vectoring Micro Controller ==
  temp_FZ : Inport  PortDimensions=[1 4]
  ang_accel : Inport  Port=2  PortDimensions=1
  acceleration : Inport  Port=3
  driver_input : Inport  Port=4  PortDimensions=1
  V : Inport  Port=5  PortDimensions=[1 2]
  yaw : Inport  Port=6  PortDimensions=1
  power_limits : Inport  Port=7  PortDimensions=[1 2]
  steering_angle : Inport  Port=8  PortDimensions=[1 2]
  brake_pressure : Inport  Port=9  PortDimensions=[1 4]
  omega : Inport  Port=10  PortDimensions=[1 4]
  shock_displacement : Inport  Port=11  PortDimensions=[1 4]
  shock_velocity : Inport  Port=12  PortDimensions=[1 4]
  previous_Tx : Inport  Port=13  PortDimensions=[1 4]
  Brake Model : MATLAB Function  TreatAsAtomicUnit=on
  Constraint Generation : MATLAB Function  TreatAsAtomicUnit=on
  Demux : Demux  Outputs=2
  Demux1 : Demux
  Divide : Product  Inputs=*/
  Divide1 : Product  Inputs=*/
  Divide3 : Product  Inputs=*/
  Mux1 : Mux  Inputs=2
  Mux2 : Mux  Inputs=2
  Normal Force Model : MATLAB Function  TreatAsAtomicUnit=on
  PIT Controller : Subsystem
  Reference Generation : MATLAB Function  TreatAsAtomicUnit=on
  Steering Model : MATLAB Function  TreatAsAtomicUnit=on
  Sum : Sum  Inputs=+
  Terminator{,1..3,6} (5 alike) : Terminator
  Tire Model : MATLAB Function  TreatAsAtomicUnit=on
  Unit Delay{,1,3..4} (4 alike) : UnitDelay  SampleTime=-1  HasFrameUpgradeWarning=on
  di : Outport  PortDimensions=1
  b : Outport  Port=2
  beq : Outport  Port=3
  lb : Outport  Port=4
  ub : Outport  Port=5
  prev_Tx : Outport  Port=6  PortDimensions=[1 4]
  Aeq : Outport  Port=7
  omega_m : Outport  Port=8  PortDimensions=[1 4]
  A : Outport  Port=9
  wires:
  temp_FZ/1 -> Normal Force Model/1(temp_FZ)  "FZ"
  Normal Force Model/1(FZ) -> Tire Model/1(FZ)
  [velocity] -> Brake Model/2(V)
  shock_displacement/1 -> [shock_d]
  shock_velocity/1 -> [shock_v]
  [shock_v] -> Normal Force Model/3(shock_velocity)
  [shock_d] -> Normal Force Model/2(shock_displacement)
  V/1 -> [velocity]  "V"
  [velocity] -> Reference Generation/2(V)
  Reference Generation/1(reference_yaw) -> PIT Controller/1(reference_yaw)
  yaw/1 -> [yaw]  "Yaw"
  [yaw] -> PIT Controller/2(yaw)
  ang_accel/1 -> [ang_accel]
  [ang_accel] -> PIT Controller/3(Angular Acceleration)
  [windup] -> PIT Controller/4(windup)
  [velocity] -> Tire Model/2(V)
  [yaw] -> Tire Model/3(yaw)
  [omega] -> Tire Model/4(omega)
  power_limits/1 -> [power_limits]
  [previous_Tx] -> Constraint Generation/1(previous_Tx)
  [driver_input] -> Constraint Generation/2(driver_input)
  [power_limits] -> Constraint Generation/3(power_limits_battery)
  Tire Model/1(Fx_max) -> Constraint Generation/6(Fx_max)
  Tire Model/2(FY) -> Constraint Generation/7(FY)
  PIT Controller/1(Control Signal) -> Constraint Generation/9(control_signal)  "Control Signal"
  Brake Model/1(T_brake) -> Constraint Generation/8(T_brake)
  [omega] -> Sum/1, Constraint Generation/4(omega)
  Steering Model/1(steering) -> [steering]
  [control_steering] -> Reference Generation/1(steering_angles)
  [steering] -> Tire Model/5(steering)
  [steering] -> Constraint Generation/5(steering)
  [target_ang_accel] -> PIT Controller/5(target_angular_acceleration)
  Unit Delay/1 -> [windup]
  Constraint Generation/10(windup) -> Unit Delay/1
  Unit Delay1/1 -> [target_ang_accel]
  Constraint Generation/9(target_ang_accel) -> Unit Delay1/1
  Constraint Generation/8(y) -> [y]
  Unit Delay3/1 -> [prev_plb]
  Constraint Generation/11(power_limit_battery) -> Unit Delay3/1
  Constraint Generation/12(integrator_reset) -> Unit Delay4/1
  Unit Delay4/1 -> [reset]
  [prev_plb] -> Constraint Generation/10(prev_plb)
  [reset] -> PIT Controller/6(reset)
  brake_pressure/1 -> [brake_pressure]  "brake_pressure"
  [brake_pressure] -> Brake Model/1(brake_pressure)
  acceleration/1 -> [acceleration]
  Constraint Generation/7(beq) -> beq/1
  Constraint Generation/5(b) -> Divide/1, b/1
  Constraint Generation/2(lb) -> lb/1
  [previous_Tx] -> prev_Tx/1
  [driver_input] -> di/1
  [omega_m] -> omega_m/1
  Constraint Generation/6(Aeq) -> Aeq/1
  Constraint Generation/4(A) -> A/1
  Constraint Generation/13(omega_m) -> [omega_m]
  previous_Tx/1 -> [previous_Tx]
  Constraint Generation/3(ub) -> ub/1
  Constraint Generation/1(power_limit) -> Terminator/1
  omega/1 -> [omega]
  Sum/1 -> Divide/2
  Divide/1 -> Terminator1/1
  driver_input/1 -> [driver_input]  "driver_input"
  steering_angle/1 -> Demux/1
  Demux/1 -> Steering Model/1(steering_angle), [control_steering]
  Demux/2 -> Terminator2/1
  Tire Model/3(FX) -> Divide1/1, Terminator3/1
  [previous_Tx] -> Divide1/2
  Demux1/3 -> Mux2/1
  Demux1/1 -> Mux1/1
  Demux1/2 -> Mux1/2
  Demux1/4 -> Mux2/2
  Divide3/1 -> Terminator6/1
  Mux2/1 -> Divide3/1
  Divide1/1 -> Demux1/1
  Mux1/1 -> Divide3/2

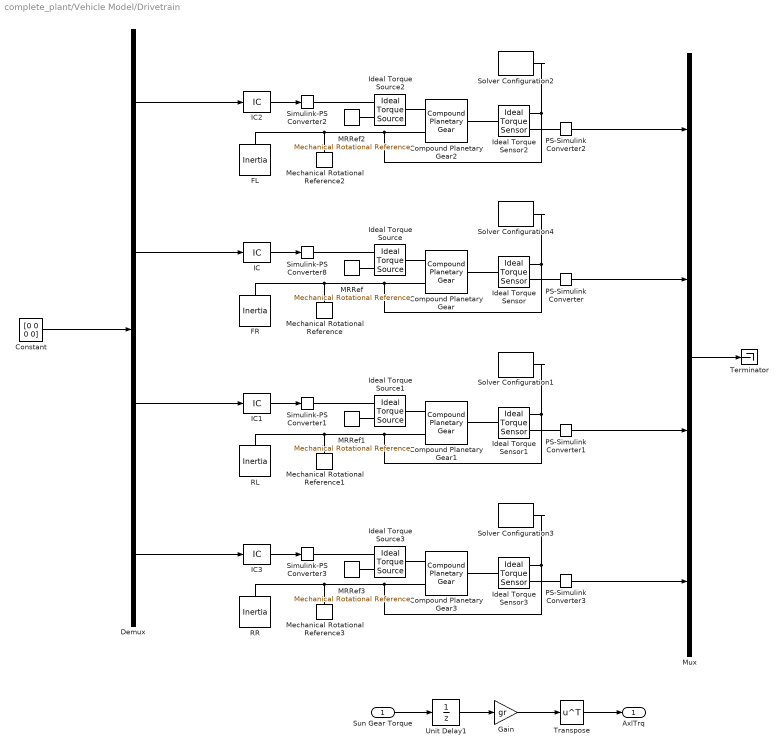
== system complete_plant/Vehicle Model/Drivetrain ==
  Sun Gear Torque : Inport
  Compound Planetary Gear : sdl_lib/Gears/Compound Planetary Gear  rp_ratio=84/23  ps_ratio=37/24  friction_model=sdl.enum.gear_friction.constant  efficiency=[.97, 1]  temperature_TLU=[280, 300, 320] K  efficiency_sp_TLU=[.95, .9, .85]  efficiency_rp_TLU=[.95, .9, .85]  pwr_thr=[.001, .001] W  mu_visc=[0, 0] N*m/(rad/s)  model_inertia=simscape.enum.onoff.off  planet_inertia=0.001 kg*m^2  thermal_mass=50 J/K  T_init=300 K
      settings: SourceProductBaseCode=LD  InternalSimscapePortConfiguration="{\"Bottom\":[],\"Left\":[{\"id\":\"C\",\"label\":\"C\",\"type\":\"foundation.mechanical.rotational.rotational\"}],\"Right\":[{\"id\":\"R\",\"label\":\"R\",\"type\":\"foundation.mechanical.rotational.rotational\"},{\"id\":\"S\",\"label\":\"S\",\"type\":\"foundation.mechanical.rotational.rotational\"}],\"Top\":[]}"
  Compound Planetary Gear1 : sdl_lib/Gears/Compound Planetary Gear  rp_ratio=84/23  ps_ratio=40/21  friction_model=sdl.enum.gear_friction.constant  efficiency=[.97, 1]  temperature_TLU=[280, 300, 320] K  efficiency_sp_TLU=[.95, .9, .85]  efficiency_rp_TLU=[.95, .9, .85]  pwr_thr=[.001, .001] W  mu_visc=[0, 0] N*m/(rad/s)  model_inertia=simscape.enum.onoff.off  planet_inertia=0.001 kg*m^2  thermal_mass=50 J/K  T_init=300 K
      settings: SourceProductBaseCode=LD  InternalSimscapePortConfiguration="{\"Bottom\":[],\"Left\":[{\"id\":\"C\",\"label\":\"C\",\"type\":\"foundation.mechanical.rotational.rotational\"}],\"Right\":[{\"id\":\"R\",\"label\":\"R\",\"type\":\"foundation.mechanical.rotational.rotational\"},{\"id\":\"S\",\"label\":\"S\",\"type\":\"foundation.mechanical.rotational.rotational\"}],\"Top\":[]}"
  Compound Planetary Gear2 : sdl_lib/Gears/Compound Planetary Gear  rp_ratio=84/23  ps_ratio=37/24  friction_model=sdl.enum.gear_friction.constant  efficiency=[.97, 1]  temperature_TLU=[280, 300, 320] K  efficiency_sp_TLU=[.95, .9, .85]  efficiency_rp_TLU=[.95, .9, .85]  pwr_thr=[.001, .001] W  mu_visc=[0, 0] N*m/(rad/s)  model_inertia=simscape.enum.onoff.off  planet_inertia=0.001 kg*m^2  thermal_mass=50 J/K  T_init=300 K
      settings: SourceProductBaseCode=LD  InternalSimscapePortConfiguration="{\"Bottom\":[],\"Left\":[{\"id\":\"C\",\"label\":\"C\",\"type\":\"foundation.mechanical.rotational.rotational\"}],\"Right\":[{\"id\":\"R\",\"label\":\"R\",\"type\":\"foundation.mechanical.rotational.rotational\"},{\"id\":\"S\",\"label\":\"S\",\"type\":\"foundation.mechanical.rotational.rotational\"}],\"Top\":[]}"
  Compound Planetary Gear3 : sdl_lib/Gears/Compound Planetary Gear  rp_ratio=84/23  ps_ratio=40/21  friction_model=sdl.enum.gear_friction.constant  efficiency=[.97, 1]  temperature_TLU=[280, 300, 320] K  efficiency_sp_TLU=[.95, .9, .85]  efficiency_rp_TLU=[.95, .9, .85]  pwr_thr=[.001, .001] W  mu_visc=[0, 0] N*m/(rad/s)  model_inertia=simscape.enum.onoff.off  planet_inertia=0.001 kg*m^2  thermal_mass=50 J/K  T_init=300 K
      settings: SourceProductBaseCode=LD  InternalSimscapePortConfiguration="{\"Bottom\":[],\"Left\":[{\"id\":\"C\",\"label\":\"C\",\"type\":\"foundation.mechanical.rotational.rotational\"}],\"Right\":[{\"id\":\"R\",\"label\":\"R\",\"type\":\"foundation.mechanical.rotational.rotational\"},{\"id\":\"S\",\"label\":\"S\",\"type\":\"foundation.mechanical.rotational.rotational\"}],\"Top\":[]}"
  Constant : Constant  Value=[0 0 0 0]
  Demux : Demux
  FL : fl_lib/Mechanical/Rotational Elements/Inertia  inertia=0.1 kg*m^2  num_ports=foundation.enum.numPorts2.one  w_specify=off  w_priority=High  w=0 rad/s  w_nominal_specify=off  w_nominal_unit=rad/s  w_nominal_value=1  t_specify=off  t_priority=None  t=0 N*m  t_nominal_specify=off  t_nominal_unit=N*m  t_nominal_value=1
  FR : fl_lib/Mechanical/Rotational Elements/Inertia  inertia=0.1 kg*m^2  num_ports=foundation.enum.numPorts2.one  w_specify=off  w_priority=High  w=0 rad/s  w_nominal_specify=off  w_nominal_unit=rad/s  w_nominal_value=1  t_specify=off  t_priority=None  t=0 N*m  t_nominal_specify=off  t_nominal_unit=N*m  t_nominal_value=1
  Gain : Gain  Gain=gr
  IC{,1..3} (4 alike) : InitialCondition  Value=0
  Ideal Torque Sensor{,1..3} (4 alike) : fl_lib/Mechanical/Mechanical Sensors/Ideal Torque Sensor
  Ideal Torque Source{,1..3} (4 alike) : fl_lib/Mechanical/Mechanical Sources/Ideal Torque Source
      settings: SourceProductName=Foundation Library
  MRRef{,1..3} (4 alike) : fl_lib/Mechanical/Rotational Elements/Mechanical Rotational Reference
      settings: SourceProductName=Foundation Library
  Mechanical Rotational Reference{,1..3} (4 alike) : fl_lib/Mechanical/Rotational Elements/Mechanical Rotational Reference
  Mux : Mux
  PS-Simulink Converter{,1..3} (4 alike) : nesl_utility/PS-Simulink Converter  PhysicalDomain=network_engine_domain  SubClassName=ps_output  LeftPortType=input  RightPortType=output  PseudoPeriodic=off  Frequencies=[]  Unit=inherit  AffineConversion=off
      settings: SourceProductBaseCode=PW,SS
  RL : fl_lib/Mechanical/Rotational Elements/Inertia  inertia=0.1 kg*m^2  num_ports=foundation.enum.numPorts2.one  w_specify=off  w_priority=High  w=0 rad/s  w_nominal_specify=off  w_nominal_unit=rad/s  w_nominal_value=1  t_specify=off  t_priority=None  t=0 N*m  t_nominal_specify=off  t_nominal_unit=N*m  t_nominal_value=1
  RR : fl_lib/Mechanical/Rotational Elements/Inertia  inertia=0.1 kg*m^2  num_ports=foundation.enum.numPorts2.one  w_specify=off  w_priority=High  w=0 rad/s  w_nominal_specify=off  w_nominal_unit=rad/s  w_nominal_value=1  t_specify=off  t_priority=None  t=0 N*m  t_nominal_specify=off  t_nominal_unit=N*m  t_nominal_value=1
  Simulink-PS Converter{1..3,8} (4 alike) : nesl_utility/Simulink-PS Converter  PhysicalDomain=network_engine_domain  SubClassName=ps_input  LeftPortType=input  RightPortType=output  PseudoPeriodic=off  Frequencies=[]  NoiseDistribution=none  NoiseParameters=[]  Unit=N*m  AffineConversion=off  FilteringAndDerivatives=zero  SimscapeFilterOrder=1  InputFilterTimeConstant=0.001  UdotUserProvided=0
      settings: SourceProductBaseCode=PW,SS
  Solver Configuration{1..4} (4 alike) : nesl_utility/Solver Configuration  PhysicalDomain=network_engine_domain  SubClassName=solver  LeftPortType=input  RightPortType=generic  Tones=[]  Harmonics=[]  SimulateNoise=off  Profile=off  UseLocalSampling=off  EnableSwitchedLinearOptims=on  FrequencyDomain=off  UseCCode=off  RelTol=0.001  AbsTol=1e-06  MinStep=1e-09  ToWorkspace=off  RevertToSquareIcSolve=off  NumHomotopyIterations=100  PhasorMode=off  PhasorModeNumHarmonics=1  DoDC=off  ResidualTolerance=1e-09  UseLocalSolver=on  LocalSolverChoice=NE_BACKWARD_EULER_ADVANCER  LocalSolverSampleTime=0.0005  DoFixedCost=off  MaxNonlinIter=300  MaxModeIter=2  ComputeImpulses=off  ImpulseIterations=2  LinearAlgebra=auto  EquationFormulation=NE_TIME_EF  DelaysMemoryBudget=1024  AutomaticFiltering=off  FilteringTimeConstant=0.001  PartitionStorageMethod=AS_NEEDED  PartitionMemoryBudget=1024  PartitionMethod=ROBUST
      settings: SourceProductBaseCode=PW,SS
  Terminator : Terminator
  Transpose : Math  Operator=transpose  SaturateOnIntegerOverflow=on
  Unit Delay1 : UnitDelay  InitialCondition=[0 0 0 0]  SampleTime=0.0005  HasFrameUpgradeWarning=on
  AxlTrq : Outport
  wires:
  IC/1 -> Simulink-PS Converter8/1
  Sun Gear Torque/1 -> Unit Delay1/1
  IC1/1 -> Simulink-PS Converter1/1
  IC2/1 -> Simulink-PS Converter2/1
  IC3/1 -> Simulink-PS Converter3/1
  Demux/1 -> IC2/1
  Demux/4 -> IC3/1
  Demux/3 -> IC1/1
  Demux/2 -> IC/1
  PS-Simulink Converter2/1 -> Mux/1
  PS-Simulink Converter3/1 -> Mux/4
  PS-Simulink Converter1/1 -> Mux/3
  PS-Simulink Converter/1 -> Mux/2
  Constant/1 -> Demux/1
  Mux/1 -> Terminator/1
  Unit Delay1/1 -> Gain/1
  Transpose/1 -> AxlTrq/1
  Gain/1 -> Transpose/1
  connections:
  MRRef/LConn1 -- Ideal Torque Source/RConn2
  FR/LConn1 -- Compound Planetary Gear/RConn1 -- Solver Configuration4/RConn1 -- Ideal Torque Sensor/RConn1 -- Mechanical Rotational Reference/LConn1
  Compound Planetary Gear/RConn2 -- Ideal Torque Source/LConn1
  Ideal Torque Source/RConn1 -- Simulink-PS Converter8/RConn1
  Compound Planetary Gear/LConn1 -- Ideal Torque Sensor/LConn1
  PS-Simulink Converter/LConn1 -- Ideal Torque Sensor/RConn2
  Ideal Torque Sensor1/RConn1 -- Mechanical Rotational Reference1/LConn1 -- RL/LConn1 -- Compound Planetary Gear1/RConn1 -- Solver Configuration1/RConn1
  Ideal Torque Source1/RConn1 -- Simulink-PS Converter1/RConn1
  Compound Planetary Gear1/RConn2 -- Ideal Torque Source1/LConn1
  PS-Simulink Converter1/LConn1 -- Ideal Torque Sensor1/RConn2
  MRRef1/LConn1 -- Ideal Torque Source1/RConn2
  Ideal Torque Sensor1/LConn1 -- Compound Planetary Gear1/LConn1
  Ideal Torque Sensor2/RConn1 -- Compound Planetary Gear2/RConn1 -- Mechanical Rotational Reference2/LConn1 -- FL/LConn1 -- Solver Configuration2/RConn1
  Ideal Torque Source2/RConn1 -- Simulink-PS Converter2/RConn1
  MRRef2/LConn1 -- Ideal Torque Source2/RConn2
  Compound Planetary Gear2/RConn2 -- Ideal Torque Source2/LConn1
  PS-Simulink Converter2/LConn1 -- Ideal Torque Sensor2/RConn2
  Compound Planetary Gear2/LConn1 -- Ideal Torque Sensor2/LConn1
  Ideal Torque Sensor3/RConn1 -- Mechanical Rotational Reference3/LConn1 -- RR/LConn1 -- Compound Planetary Gear3/RConn1 -- Solver Configuration3/RConn1
  Compound Planetary Gear3/RConn2 -- Ideal Torque Source3/LConn1
  Ideal Torque Sensor3/LConn1 -- Compound Planetary Gear3/LConn1
  MRRef3/LConn1 -- Ideal Torque Source3/RConn2
  PS-Simulink Converter3/LConn1 -- Ideal Torque Sensor3/RConn2
  Ideal Torque Source3/RConn1 -- Simulink-PS Converter3/RConn1
